simulink model "simple_switch1"  (R2023b)
settings: Solver=VariableStepAuto  StartTime=0.0  StopTime=50  RelTol=1e-3
undefined symbols (not defined in the file): csd_100
settings Model: Creator=39216  LastModifiedBy=39216

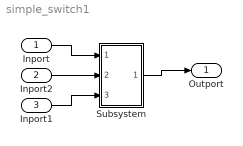
== system simple_switch1 ==
  Inport : Inport
  Inport2 : Inport  Port=2
  Inport1 : Inport  Port=3
  Subsystem : Subsystem
  Outport : Outport
  wires:
  Subsystem/1(Outport) -> Outport/1
  Inport/1 -> Subsystem/1(Inport)
  Inport1/1 -> Subsystem/3(Inport1)
  Inport2/1 -> Subsystem/2(Inport2)

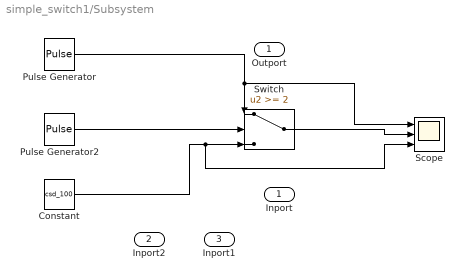
== system simple_switch1/Subsystem ==
  Inport : Inport
  Inport2 : Inport  Port=2
  Inport1 : Inport  Port=3
  Constant : Constant  Value=csd_100
  Pulse Generator : DiscretePulseGenerator  PulseType=Time based  Period=10  PulseWidth=50
  Pulse Generator2 : DiscretePulseGenerator  PulseType=Time based  Period=10  PulseWidth=5
  Scope : Scope  NumInputPorts=3
  Switch : Switch  Threshold=2  SaturateOnIntegerOverflow=off  InputSameDT=off
  Outport : Outport
  wires:
  Pulse Generator/1 -> Scope/1, Switch/1
  Switch/1 -> Scope/2
  Constant/1 -> Scope/3, Switch/3
  Pulse Generator2/1 -> Switch/2
